simulink library "LeafEcoTronDBWLib"  (R2018a)
settings: Solver=VariableStepAuto  StartTime=0.0  StopTime=10.0  RelTol=1e-3
libraries: Simulink x17, CoderSF_BSW_Libs x3
(part 1 of 2)
settings Model: Creator=TianhuaZhang  LastModifiedBy=TianhuaZhang

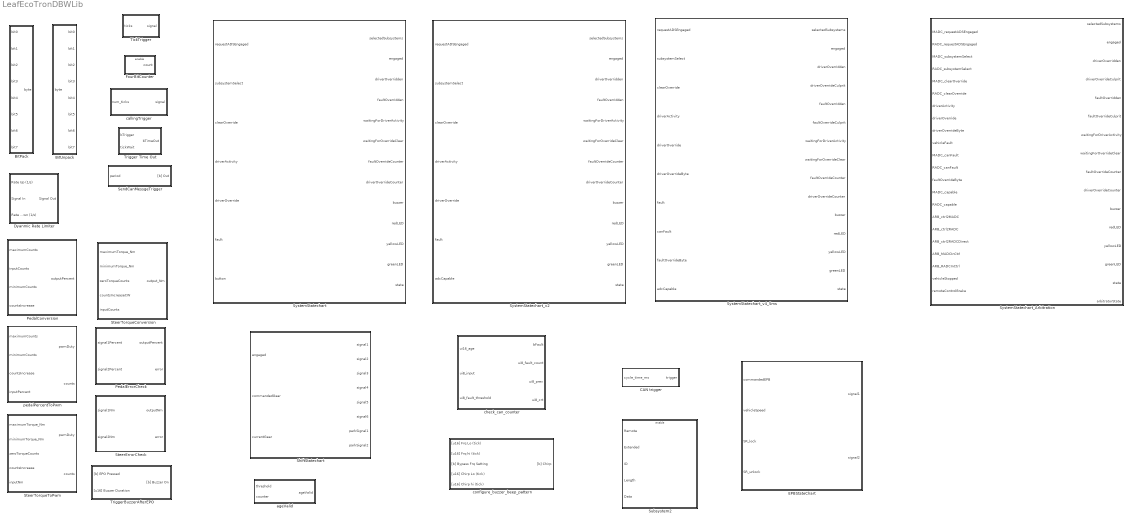
== system LeafEcoTronDBWLib ==
  BitPack : Subsystem
  BitUnpack : Subsystem
  CAN trigger : Subsystem
  Dyanmic Rate Limiter : Subsystem
  EPBStateChart : Stateflow chart  TreatAsAtomicUnit=on
  FourBitCounter : Subsystem
  PedalConversion : Subsystem
  PedalErrorCheck : Subsystem
  SendCanMessgeTrigger : Subsystem
  ShiftStatechart : Stateflow chart  TreatAsAtomicUnit=on
  SteerErrorCheck : Subsystem
  SteerTorqueConversion : Subsystem
  SteerTorqueToPwm : Subsystem
  Subsystem2 : Subsystem
  SystemStatechart : Stateflow chart  TreatAsAtomicUnit=on
  SystemStatechart_Arbitration : Stateflow chart  TreatAsAtomicUnit=on
  SystemStatechart_v2 : Stateflow chart  TreatAsAtomicUnit=on
  SystemStatechart_v4_5ms : Stateflow chart  TreatAsAtomicUnit=on
  TickTrigger : Subsystem
  Trigger Time Out : Subsystem
  TriggerBuzzerAfterEPO : Subsystem
      settings: AttributesFormatString=%<ReferenceBlock>
  ageValid : Subsystem
  callingTrigger : MATLAB Function  TreatAsAtomicUnit=on
  check_can_counter : Stateflow chart  TreatAsAtomicUnit=on
      settings: AttributesFormatString=%<ReferenceBlock>
  configure_buzzer_beep_pattern : Subsystem
      settings: AttributesFormatString=%<ReferenceBlock>
  pedalPercentToPwm : Subsystem

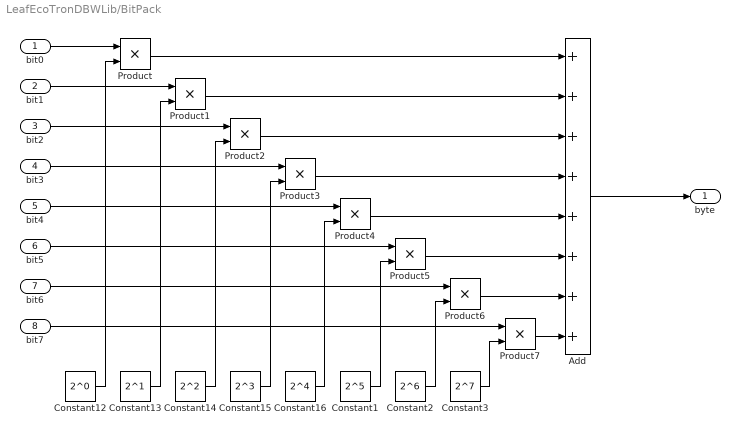
== system LeafEcoTronDBWLib/BitPack ==
  bit0 : Inport
  bit1 : Inport  Port=2
  bit2 : Inport  Port=3
  bit3 : Inport  Port=4
  bit4 : Inport  Port=5
  bit5 : Inport  Port=6
  bit6 : Inport  Port=7
  bit7 : Inport  Port=8
  Add : Sum  Inputs=++++++++  AccumDataTypeStr=uint8  OutDataTypeStr=uint8
  Constant1 : Constant  Value=2^5  OutDataTypeStr=uint8
  Constant12 : Constant  Value=2^0  OutDataTypeStr=uint8
  Constant13 : Constant  Value=2^1  OutDataTypeStr=uint8
  Constant14 : Constant  Value=2^2  OutDataTypeStr=uint8
  Constant15 : Constant  Value=2^3  OutDataTypeStr=uint8
  Constant16 : Constant  Value=2^4  OutDataTypeStr=uint8
  Constant2 : Constant  Value=2^6  OutDataTypeStr=uint8
  Constant3 : Constant  Value=2^7  OutDataTypeStr=uint8
  Product : Product  OutDataTypeStr=int16
  Product{1..7} (7 alike) : Product  OutDataTypeStr=uint8
  byte : Outport
  wires:
  Constant3/1 -> Product7/2
  Constant2/1 -> Product6/2
  Constant1/1 -> Product5/2
  Product6/1 -> Add/7
  Product5/1 -> Add/6
  bit5/1 -> Product5/1
  bit6/1 -> Product6/1
  bit7/1 -> Product7/1
  Product7/1 -> Add/8
  Product1/1 -> Add/2
  Product/1 -> Add/1
  Product4/1 -> Add/5
  Add/1 -> byte/1
  Constant16/1 -> Product4/2
  Product3/1 -> Add/4
  bit0/1 -> Product/1
  bit1/1 -> Product1/1
  bit3/1 -> Product3/1
  Constant13/1 -> Product1/2
  bit4/1 -> Product4/1
  Constant14/1 -> Product2/2
  bit2/1 -> Product2/1
  Constant15/1 -> Product3/2
  Constant12/1 -> Product/2
  Product2/1 -> Add/3

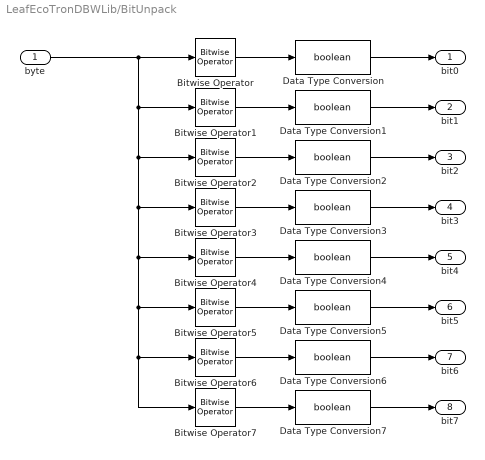
== system LeafEcoTronDBWLib/BitUnpack ==
  byte : Inport
  Bitwise Operator : Simulink/Logic and Bit Operations/Bitwise Operator  logicop=AND  UseBitMask=on  BitMask=2^0  BitMaskRealWorld=Stored Integer
      settings: SourceProductName=Simulink  SourceProductBaseCode=SL
  Bitwise Operator1 : Simulink/Logic and Bit Operations/Bitwise Operator  logicop=AND  UseBitMask=on  BitMask=2^1  BitMaskRealWorld=Stored Integer
      settings: SourceProductName=Simulink  SourceProductBaseCode=SL
  Bitwise Operator2 : Simulink/Logic and Bit Operations/Bitwise Operator  logicop=AND  UseBitMask=on  BitMask=2^2  BitMaskRealWorld=Stored Integer
      settings: SourceProductName=Simulink  SourceProductBaseCode=SL
  Bitwise Operator3 : Simulink/Logic and Bit Operations/Bitwise Operator  logicop=AND  UseBitMask=on  BitMask=2^3  BitMaskRealWorld=Stored Integer
      settings: SourceProductName=Simulink  SourceProductBaseCode=SL
  Bitwise Operator4 : Simulink/Logic and Bit Operations/Bitwise Operator  logicop=AND  UseBitMask=on  BitMask=2^4  BitMaskRealWorld=Stored Integer
      settings: SourceProductName=Simulink  SourceProductBaseCode=SL
  Bitwise Operator5 : Simulink/Logic and Bit Operations/Bitwise Operator  logicop=AND  UseBitMask=on  BitMask=2^5  BitMaskRealWorld=Stored Integer
      settings: SourceProductName=Simulink  SourceProductBaseCode=SL
  Bitwise Operator6 : Simulink/Logic and Bit Operations/Bitwise Operator  logicop=AND  UseBitMask=on  BitMask=2^6  BitMaskRealWorld=Stored Integer
      settings: SourceProductName=Simulink  SourceProductBaseCode=SL
  Bitwise Operator7 : Simulink/Logic and Bit Operations/Bitwise Operator  logicop=AND  UseBitMask=on  BitMask=2^7  BitMaskRealWorld=Stored Integer
      settings: SourceProductName=Simulink  SourceProductBaseCode=SL
  Data Type Conversion{,1..7} (8 alike) : DataTypeConversion  OutDataTypeStr=boolean
  bit0 : Outport
  bit1 : Outport  Port=2
  bit2 : Outport  Port=3
  bit3 : Outport  Port=4
  bit4 : Outport  Port=5
  bit5 : Outport  Port=6
  bit6 : Outport  Port=7
  bit7 : Outport  Port=8
  wires:
  Data Type Conversion7/1 -> bit7/1
  Data Type Conversion6/1 -> bit6/1
  Data Type Conversion5/1 -> bit5/1
  Data Type Conversion4/1 -> bit4/1
  Data Type Conversion3/1 -> bit3/1
  Data Type Conversion2/1 -> bit2/1
  Data Type Conversion1/1 -> bit1/1
  Data Type Conversion/1 -> bit0/1
  Bitwise Operator7/1 -> Data Type Conversion7/1
  Bitwise Operator6/1 -> Data Type Conversion6/1
  Bitwise Operator5/1 -> Data Type Conversion5/1
  Bitwise Operator4/1 -> Data Type Conversion4/1
  Bitwise Operator3/1 -> Data Type Conversion3/1
  Bitwise Operator2/1 -> Data Type Conversion2/1
  Bitwise Operator1/1 -> Data Type Conversion1/1
  byte/1 -> Bitwise Operator/1, Bitwise Operator7/1, Bitwise Operator6/1, Bitwise Operator5/1, Bitwise Operator4/1, Bitwise Operator3/1, Bitwise Operator2/1, Bitwise Operator1/1
  Bitwise Operator/1 -> Data Type Conversion/1

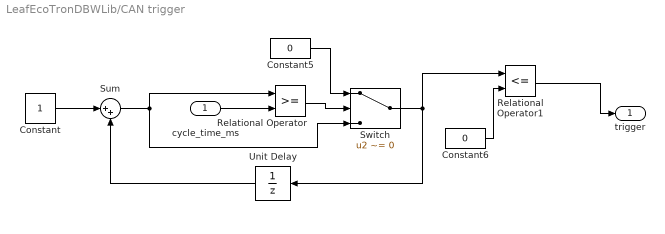
== system LeafEcoTronDBWLib/CAN trigger ==
  cycle_time_ms : Inport
  Constant : Constant  OutDataTypeStr=Inherit: Inherit via back propagation
  Constant5 : Constant  Value=0  OutDataTypeStr=Inherit: Inherit via back propagation  SampleTime=-1
  Constant6 : Constant  Value=0  OutDataTypeStr=Inherit: Inherit via back propagation  SampleTime=-1
  Relational Operator : RelationalOperator  OutDataTypeStr=boolean  RndMeth=Nearest
  Relational Operator1 : RelationalOperator  Operator=<=  OutDataTypeStr=boolean  RndMeth=Nearest
  Sum : Sum  Inputs=|++
  Switch : Switch  Criteria=u2 ~= 0
  Unit Delay : UnitDelay  SampleTime=-1
  trigger : Outport
  wires:
  cycle_time_ms/1 -> Relational Operator/2
  Relational Operator1/1 -> trigger/1
  Unit Delay/1 -> Sum/2
  Constant/1 -> Sum/1
  Relational Operator/1 -> Switch/2
  Constant5/1 -> Switch/1
  Switch/1 -> Relational Operator1/1, Unit Delay/1
  Sum/1 -> Switch/3, Relational Operator/1
  Constant6/1 -> Relational Operator1/2

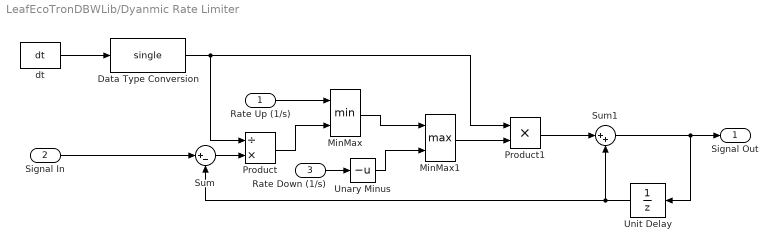
== system LeafEcoTronDBWLib/Dyanmic Rate Limiter ==
  Rate Up (1/s) : Inport
  Signal In : Inport  Port=2
  Rate Down (1/s) : Inport  Port=3
  Data Type Conversion : DataTypeConversion  OutDataTypeStr=single
  MinMax : MinMax  Inputs=2
  MinMax1 : MinMax  Function=max  Inputs=2
  Product : Product  Inputs=/*  RndMeth=Zero
  Product1 : Product  RndMeth=Zero
  Sum : Sum  Inputs=|+-
  Sum1 : Sum  Inputs=|++
  Unary Minus : UnaryMinus
  Unit Delay : UnitDelay  SampleTime=-1
  dt : CoderSF_BSW_Libs/Application Base Blocks/dt
      settings: SourceProductName=EcoCoder Blocks
  Signal Out : Outport  OutDataTypeStr=single
  wires:
  dt/1 -> Data Type Conversion/1
  Rate Up (1/s)/1 -> MinMax/1
  MinMax/1 -> MinMax1/1
  Rate Down (1/s)/1 -> Unary Minus/1
  Product/1 -> MinMax/2
  Data Type Conversion/1 -> Product/1, Product1/1
  Sum/1 -> Product/2
  MinMax1/1 -> Product1/2
  Product1/1 -> Sum1/1
  Unit Delay/1 -> Sum1/2, Sum/2
  Sum1/1 -> Unit Delay/1, Signal Out/1
  Signal In/1 -> Sum/1
  Unary Minus/1 -> MinMax1/2

== system LeafEcoTronDBWLib/FourBitCounter ==
  Enable : EnablePort
  Counter Limited : Simulink/Sources/Counter Limited  uplimit=15  tsamp=-1
      settings: SourceProductName=Simulink  SourceProductBaseCode=SL
  count : Outport
  wires:
  Counter Limited/1 -> count/1

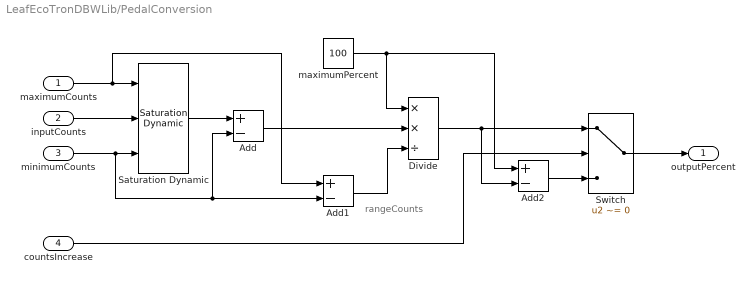
== system LeafEcoTronDBWLib/PedalConversion ==
  note: rangeCounts
  maximumCounts : Inport  OutDataTypeStr=uint16
  inputCounts : Inport  Port=2  OutDataTypeStr=uint16
  minimumCounts : Inport  Port=3  OutDataTypeStr=uint16
  countsIncrease : Inport  Port=4  OutDataTypeStr=boolean
  Add : Sum  Inputs=+-  OutDataTypeStr=single
  Add1 : Sum  Inputs=+-  OutDataTypeStr=single
  Add2 : Sum  Inputs=+-  OutDataTypeStr=single
  Divide : Product  Inputs=**/  OutDataTypeStr=single
  Saturation Dynamic : Simulink/Discontinuities/Saturation Dynamic  OutMin=[]  OutMax=[]  OutDataTypeStr=Inherit: Same as second input  OutDataType=fixdt(1, 16)  OutScaling=2^-10  DoSatur=off
      settings: SourceProductName=Simulink  SourceProductBaseCode=SL
  Switch : Switch  Criteria=u2 ~= 0
  maximumPercent : Constant  Value=100  OutDataTypeStr=single
  outputPercent : Outport
  wires:
  inputCounts/1 -> Saturation Dynamic/2
  Add1/1 -> Divide/3
  maximumPercent/1 -> Add2/1, Divide/1
  Add/1 -> Divide/2
  minimumCounts/1 -> Add/2, Add1/2, Saturation Dynamic/3
  maximumCounts/1 -> Add1/1, Saturation Dynamic/1
  Saturation Dynamic/1 -> Add/1
  Switch/1 -> outputPercent/1
  Divide/1 -> Add2/2, Switch/1
  countsIncrease/1 -> Switch/2
  Add2/1 -> Switch/3

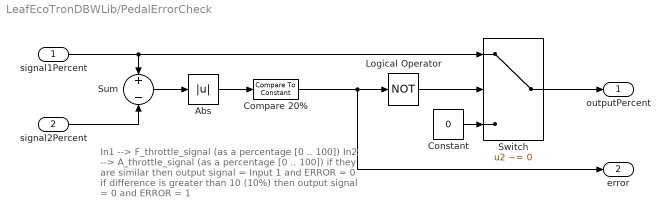
== system LeafEcoTronDBWLib/PedalErrorCheck ==
  note: In1 --> F_throttle_signal (as a percentage [0 .. 100])
      | In2 --> A_throttle_signal (as a percentage [0 .. 100])
      |
      | if they are similar then
      |     output signal = Input 1
      |     and ERROR = 0
      | if difference is greater than 10 (10%) then
      |     output signal =  0
      |     and ERROR = 1
  signal1Percent : Inport  OutDataTypeStr=single
  signal2Percent : Inport  Port=2  OutDataTypeStr=single
  Abs : Abs
  Compare 20% : Simulink/Logic and Bit Operations/Compare To Constant  relop=>=  const=20  OutDataTypeStr=boolean
      settings: SourceProductName=Simulink  SourceProductBaseCode=SL
  Constant : Constant  Value=0  OutDataTypeStr=single
  Logical Operator : Logic  Operator=NOT  AllPortsSameDT=off  OutDataTypeStr=boolean
  Sum : Sum  Inputs=+|-
  Switch : Switch  Criteria=u2 ~= 0  Threshold=0.5  OutMin=[0]  OutMax=[100]  OutDataTypeStr=single
  outputPercent : Outport  OutDataTypeStr=single
  error : Outport  Port=2  OutDataTypeStr=boolean
  wires:
  Logical Operator/1 -> Switch/2
  Constant/1 -> Switch/3
  Abs/1 -> Compare 20%/1
  Compare 20%/1 -> Logical Operator/1, error/1
  signal1Percent/1 -> Sum/1, Switch/1
  Sum/1 -> Abs/1
  signal2Percent/1 -> Sum/2
  Switch/1 -> outputPercent/1

== system LeafEcoTronDBWLib/SendCanMessgeTrigger ==
  period : Inport
  Data Type Conversion : DataTypeConversion  OutDataTypeStr=boolean
  Saturation : Saturate  UpperLimit=1000  LowerLimit=1
      settings: AttributesFormatString=[%<LowerLimit>,%<UpperLimit>]
  Terminator : Terminator
  trigger : Stateflow chart  TreatAsAtomicUnit=on
  "[b] Out" : Outport
  wires:
  trigger/2(counter) -> Terminator/1
  period/1 -> Saturation/1
  trigger/1(out) -> Data Type Conversion/1
  Data Type Conversion/1 -> "[b] Out"/1
  Saturation/1 -> trigger/1(period)

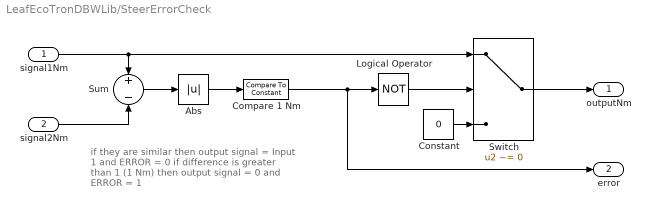
== system LeafEcoTronDBWLib/SteerErrorCheck ==
  note: if they are similar then
      |     output signal = Input 1
      |     and ERROR = 0
      | if difference is greater than 1 (1 Nm) then
      |     output signal =  0
      |     and ERROR = 1
  signal1Nm : Inport  OutDataTypeStr=single
  signal2Nm : Inport  Port=2  OutDataTypeStr=single
  Abs : Abs
  Compare 1 Nm : Simulink/Logic and Bit Operations/Compare To Constant  relop=>=  const=1  OutDataTypeStr=boolean
      settings: SourceProductName=Simulink  SourceProductBaseCode=SL
  Constant : Constant  Value=0  OutDataTypeStr=single
  Logical Operator : Logic  Operator=NOT  AllPortsSameDT=off  OutDataTypeStr=boolean
  Sum : Sum  Inputs=+|-
  Switch : Switch  Criteria=u2 ~= 0  Threshold=0.5  OutMin=[0]  OutMax=[100]  OutDataTypeStr=single
  outputNm : Outport  OutDataTypeStr=single
  error : Outport  Port=2  OutDataTypeStr=boolean
  wires:
  Logical Operator/1 -> Switch/2
  Constant/1 -> Switch/3
  Abs/1 -> Compare 1 Nm/1
  Compare 1 Nm/1 -> Logical Operator/1, error/1
  signal1Nm/1 -> Sum/1, Switch/1
  Sum/1 -> Abs/1
  signal2Nm/1 -> Sum/2
  Switch/1 -> outputNm/1

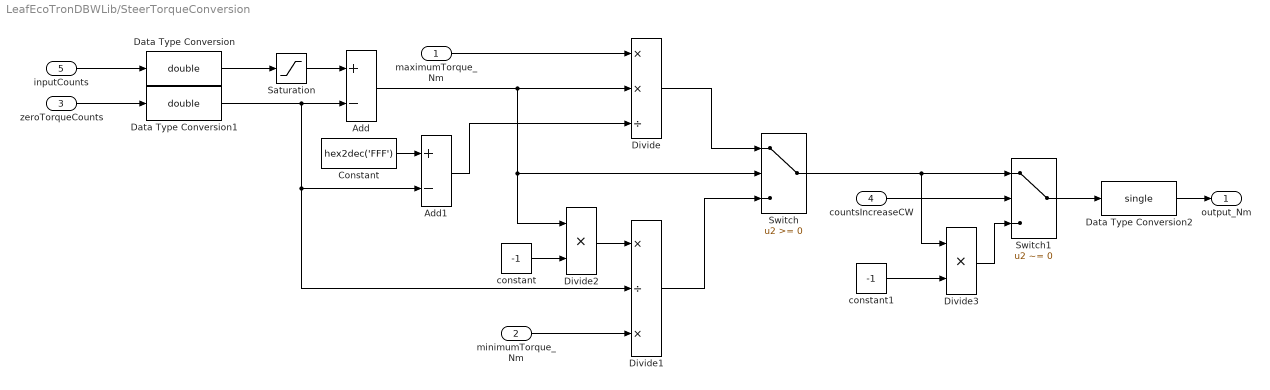
== system LeafEcoTronDBWLib/SteerTorqueConversion ==
  maximumTorque_Nm : Inport
  minimumTorque_Nm : Inport  Port=2
  zeroTorqueCounts : Inport  Port=3
  countsIncreaseCW : Inport  Port=4
  inputCounts : Inport  Port=5
  Add : Sum  Inputs=+-  OutDataTypeStr=double
  Add1 : Sum  Inputs=+-  OutDataTypeStr=double
  Constant : Constant  Value=hex2dec('FFF')  OutDataTypeStr=uint16
  Data Type Conversion : DataTypeConversion  OutDataTypeStr=double
  Data Type Conversion1 : DataTypeConversion  OutDataTypeStr=double
  Data Type Conversion2 : DataTypeConversion  OutDataTypeStr=single  LockScale=on
  Divide : Product  Inputs=**/  OutDataTypeStr=double  SaturateOnIntegerOverflow=on  RndMeth=Zero
  Divide1 : Product  Inputs=*/*  OutDataTypeStr=single  SaturateOnIntegerOverflow=on  RndMeth=Zero
  Divide2 : Product  Inputs=**  OutDataTypeStr=single  SaturateOnIntegerOverflow=on  RndMeth=Zero
  Divide3 : Product  Inputs=**  OutDataTypeStr=double  SaturateOnIntegerOverflow=on  RndMeth=Zero
  Saturation : Saturate  UpperLimit=4095  LowerLimit=0
  Switch : Switch  OutDataTypeStr=double
  Switch1 : Switch  Criteria=u2 ~= 0
  constant : Constant  Value=-1  OutDataTypeStr=single
  constant1 : Constant  Value=-1  OutDataTypeStr=single
  output_Nm : Outport
  wires:
  Data Type Conversion2/1 -> output_Nm/1
  Data Type Conversion1/1 -> Add/2, Divide1/2, Add1/2
  Data Type Conversion/1 -> Saturation/1
  Saturation/1 -> Add/1
  constant1/1 -> Divide3/2
  Divide3/1 -> Switch1/3
  countsIncreaseCW/1 -> Switch1/2
  Switch1/1 -> Data Type Conversion2/1
  Switch/1 -> Switch1/1, Divide3/1
  constant/1 -> Divide2/2
  Divide2/1 -> Divide1/1
  Divide1/1 -> Switch/3
  minimumTorque_Nm/1 -> Divide1/3
  Add1/1 -> Divide/3
  Divide/1 -> Switch/1
  maximumTorque_Nm/1 -> Divide/1
  Add/1 -> Switch/2, Divide2/1, Divide/2
  Constant/1 -> Add1/1
  zeroTorqueCounts/1 -> Data Type Conversion1/1
  inputCounts/1 -> Data Type Conversion/1

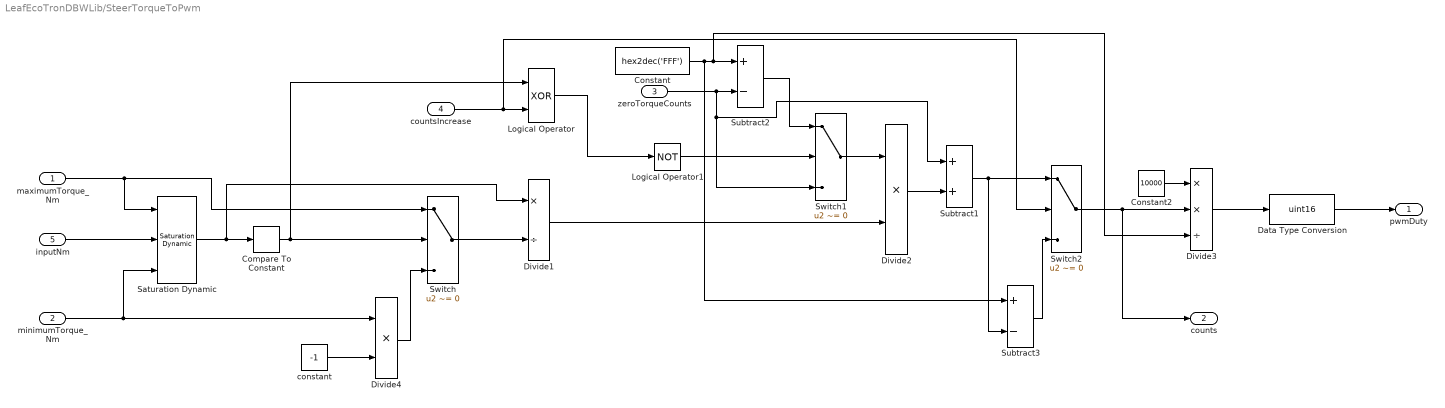
== system LeafEcoTronDBWLib/SteerTorqueToPwm ==
  maximumTorque_Nm : Inport
  minimumTorque_Nm : Inport  Port=2
  zeroTorqueCounts : Inport  Port=3
  countsIncrease : Inport  Port=4
  inputNm : Inport  Port=5
  Compare To Constant : Simulink/Logic and Bit Operations/Compare To Constant  relop=>=  const=0  OutDataTypeStr=boolean
      settings: SourceProductName=Simulink  SourceProductBaseCode=SL
  Constant : Constant  Value=hex2dec('FFF')  OutDataTypeStr=double
  Constant2 : Constant  Value=10000  OutDataTypeStr=double
  Data Type Conversion : DataTypeConversion  OutDataTypeStr=uint16
  Divide1 : Product  Inputs=*/  OutDataTypeStr=double
  Divide2 : Product  Inputs=**  OutDataTypeStr=double
  Divide3 : Product  Inputs=**/  OutDataTypeStr=double
  Divide4 : Product  Inputs=**
  Logical Operator : Logic  Operator=XOR  AllPortsSameDT=off  OutDataTypeStr=boolean
  Logical Operator1 : Logic  Operator=NOT  AllPortsSameDT=off  OutDataTypeStr=boolean
  Saturation Dynamic : Simulink/Discontinuities/Saturation Dynamic  OutMin=[]  OutMax=[]  OutDataTypeStr=Inherit: Same as second input  OutDataType=fixdt(1, 16)  OutScaling=2^-10  DoSatur=off
      settings: SourceProductName=Simulink  SourceProductBaseCode=SL
  Subtract1 : Sum  AccumDataTypeStr=double
  Subtract2 : Sum  Inputs=+-
  Subtract3 : Sum  Inputs=+-
  Switch : Switch  Criteria=u2 ~= 0  OutDataTypeStr=double
  Switch1 : Switch  Criteria=u2 ~= 0
  Switch2 : Switch  Criteria=u2 ~= 0
  constant : Constant  Value=-1  OutDataTypeStr=double
  pwmDuty : Outport
  counts : Outport  Port=2
  wires:
  Subtract3/1 -> Switch2/3
  Subtract1/1 -> Switch2/1, Subtract3/2
  Switch2/1 -> Divide3/2, counts/1
  Saturation Dynamic/1 -> Compare To Constant/1, Divide1/1
  inputNm/1 -> Saturation Dynamic/2
  Data Type Conversion/1 -> pwmDuty/1
  constant/1 -> Divide4/2
  Divide4/1 -> Switch/3
  minimumTorque_Nm/1 -> Divide4/1, Saturation Dynamic/3
  Divide2/1 -> Subtract1/2
  Logical Operator1/1 -> Switch1/2
  Logical Operator/1 -> Logical Operator1/1
  Subtract2/1 -> Switch1/1
  Compare To Constant/1 -> Logical Operator/1, Switch/2
  Divide3/1 -> Data Type Conversion/1
  Constant2/1 -> Divide3/1
  countsIncrease/1 -> Logical Operator/2, Switch2/2
  Switch1/1 -> Divide2/1
  Divide1/1 -> Divide2/2
  Switch/1 -> Divide1/2
  maximumTorque_Nm/1 -> Switch/1, Saturation Dynamic/1
  zeroTorqueCounts/1 -> Subtract2/2, Switch1/3, Subtract1/1
  Constant/1 -> Subtract2/1, Divide3/3, Subtract3/1

== system LeafEcoTronDBWLib/Subsystem2 ==
  Remote : Inport
  Extended : Inport  Port=2
  ID : Inport  Port=3
  Length : Inport  Port=4
  Data : Inport  Port=5
  Enable : EnablePort
  Transmit CAN Message : CoderSF_BSW_Libs/CAN/Transmit CAN Message  channel=CAN_B  tasktimeIndex=Task_Inherit
      settings: SourceProductName=EcoCoder Blocks
  Transmit CAN Message1 : CoderSF_BSW_Libs/CAN/Transmit CAN Message  channel=CAN_C  tasktimeIndex=Task_Inherit
      settings: SourceProductName=EcoCoder Blocks
  wires:
  Extended/1 -> Transmit CAN Message1/2, Transmit CAN Message/2
  Remote/1 -> Transmit CAN Message1/1, Transmit CAN Message/1
  Length/1 -> Transmit CAN Message1/4, Transmit CAN Message/4
  Data/1 -> Transmit CAN Message1/5, Transmit CAN Message/5
  ID/1 -> Transmit CAN Message1/3, Transmit CAN Message/3

== system LeafEcoTronDBWLib/TickTrigger ==
  ticks : Inport
  Add : Sum  OutDataTypeStr=uint8
  Compare To Zero : Simulink/Logic and Bit Operations/Compare To Zero  relop===  OutDataTypeStr=boolean
      settings: SourceProductName=Simulink  SourceProductBaseCode=SL
  Constant2 : Constant
  Memory : Memory  InheritSampleTime=on
  Mod : Math  Operator=mod  SaturateOnIntegerOverflow=on
  signal : Outport  OutDataTypeStr=boolean
  wires:
  Compare To Zero/1 -> signal/1
  Add/1 -> Mod/1
  Memory/1 -> Add/1
  Constant2/1 -> Add/2
  ticks/1 -> Mod/2
  Mod/1 -> Memory/1, Compare To Zero/1

== system LeafEcoTronDBWLib/Trigger Time Out ==
  note: -Once the bTrigger signal is high, program starts counting and set bTimeOut to high when it exceeds the tickWati
      | -bTimeOut resets as soon as bTrigger resets
  bTrigger : Inport
  tickWait : Inport  Port=2
  Constant : Constant  Value=0  OutDataTypeStr=single
      settings: AttributesFormatString=%<OutDataTypeStr>
  IC1 : InitialCondition
  Increment Real World1 : Simulink/Additional Math & Discrete/Additional Math: Increment - Decrement/Increment Real World
      settings: SourceProductName=Simulink  SourceProductBaseCode=SL
  Memory1 : Memory  InheritSampleTime=on
  Relational Operator1 : RelationalOperator  Operator=>  OutDataTypeStr=boolean  RndMeth=Nearest
  Switch1 : Switch  Criteria=u2 > Threshold
  bTimeOut : Outport
  wires:
  Relational Operator1/1 -> bTimeOut/1
  tickWait/1 -> Relational Operator1/2
  Memory1/1 -> IC1/1, Relational Operator1/1
  Switch1/1 -> Memory1/1
  Increment Real World1/1 -> Switch1/1
  IC1/1 -> Increment Real World1/1
  bTrigger/1 -> Switch1/2
  Constant/1 -> Switch1/3

== system LeafEcoTronDBWLib/TriggerBuzzerAfterEPO ==
  "[b] EPO Pressed" : Inport
  "[u16] Buzzer Duration" : Inport  Port=2
  Detect Increase : Simulink/Logic and Bit Operations/Detect Increase  vinit=0.0  OutDataTypeStr=boolean
      settings: SourceProductName=Simulink  SourceProductBaseCode=SL
  trigger_buzzer_after_epo : Stateflow chart  TreatAsAtomicUnit=on
  "[b] Buzzer On" : Outport
  wires:
  Detect Increase/1 -> trigger_buzzer_after_epo/1(bEPO_rise)
  "[b] EPO Pressed"/1 -> Detect Increase/1
  "[u16] Buzzer Duration"/1 -> trigger_buzzer_after_epo/2(tick_duration)
  trigger_buzzer_after_epo/1(bBuzzer) -> "[b] Buzzer On"/1

== system LeafEcoTronDBWLib/ageValid ==
  threshold : Inport
  counter : Inport  Port=2
  Data Type Conversion : DataTypeConversion  OutDataTypeStr=uint16
  Data Type Conversion2 : DataTypeConversion  OutDataTypeStr=boolean
  Delay : Delay  DelayLength=1
  Relational Operator : RelationalOperator  Operator=~=  OutDataTypeStr=boolean  RndMeth=Nearest
  trigger : Stateflow chart  AncestorBlock=LeafDbWLibrary/SendCanMessgeTrigger/trigger  TreatAsAtomicUnit=on
  ageValid : Outport  OutDataTypeStr=boolean
  wires:
  Delay/1 -> Relational Operator/1
  Relational Operator/1 -> trigger/2(update)
  threshold/1 -> Data Type Conversion/1
  trigger/1(ageValid) -> Data Type Conversion2/1
  Data Type Conversion/1 -> trigger/1(threshold)
  counter/1 -> Delay/1, Relational Operator/2
  Data Type Conversion2/1 -> ageValid/1

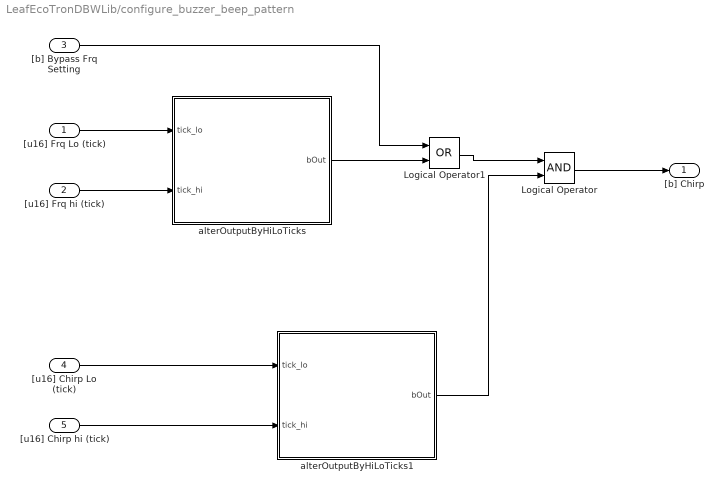
== system LeafEcoTronDBWLib/configure_buzzer_beep_pattern ==
  "[u16] Frq Lo (tick)" : Inport
  "[u16] Frq hi (tick)" : Inport  Port=2
  "[b] Bypass Frq Setting" : Inport  Port=3
  "[u16] Chirp Lo (tick)" : Inport  Port=4
  "[u16] Chirp hi (tick)" : Inport  Port=5
  Logical Operator : Logic  AllPortsSameDT=off  OutDataTypeStr=boolean
  Logical Operator1 : Logic  Operator=OR  AllPortsSameDT=off  OutDataTypeStr=boolean
  alterOutputByHiLoTicks : Stateflow chart  TreatAsAtomicUnit=on
  alterOutputByHiLoTicks1 : Stateflow chart  TreatAsAtomicUnit=on
  "[b] Chirp" : Outport
  wires:
  "[u16] Frq hi (tick)"/1 -> alterOutputByHiLoTicks/2(tick_hi)
  "[u16] Frq Lo (tick)"/1 -> alterOutputByHiLoTicks/1(tick_lo)
  "[u16] Chirp hi (tick)"/1 -> alterOutputByHiLoTicks1/2(tick_hi)
  "[u16] Chirp Lo (tick)"/1 -> alterOutputByHiLoTicks1/1(tick_lo)
  Logical Operator1/1 -> Logical Operator/1
  alterOutputByHiLoTicks1/1(bOut) -> Logical Operator/2
  Logical Operator/1 -> "[b] Chirp"/1
  alterOutputByHiLoTicks/1(bOut) -> Logical Operator1/2
  "[b] Bypass Frq Setting"/1 -> Logical Operator1/1

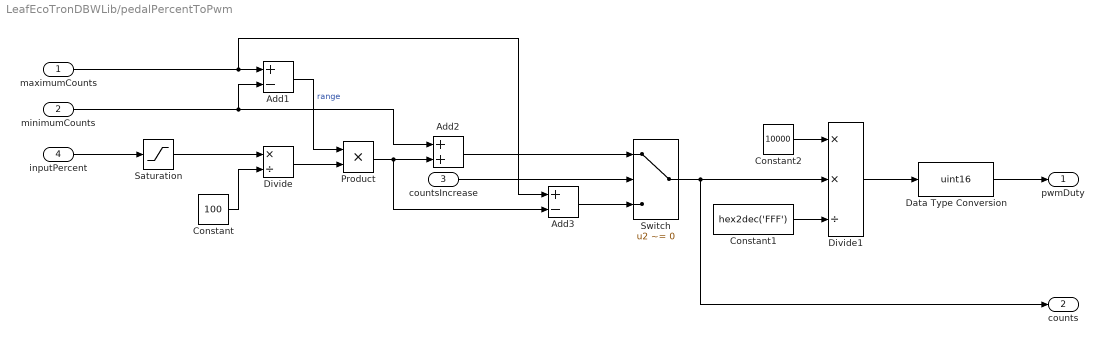
== system LeafEcoTronDBWLib/pedalPercentToPwm ==
  maximumCounts : Inport
  minimumCounts : Inport  Port=2
  countsIncrease : Inport  Port=3
  inputPercent : Inport  Port=4
  Add1 : Sum  Inputs=+-  OutDataTypeStr=single
  Add2 : Sum  OutDataTypeStr=single
  Add3 : Sum  Inputs=+-  OutDataTypeStr=single
  Constant : Constant  Value=100  OutDataTypeStr=single
  Constant1 : Constant  Value=hex2dec('FFF')  OutDataTypeStr=single
  Constant2 : Constant  Value=10000  OutDataTypeStr=single
  Data Type Conversion : DataTypeConversion  OutDataTypeStr=uint16
  Divide : Product  Inputs=*/
  Divide1 : Product  Inputs=**/  OutDataTypeStr=single
  Product : Product
  Saturation : Saturate  UpperLimit=100.0  LowerLimit=0.0
  Switch : Switch  Criteria=u2 ~= 0
  pwmDuty : Outport
  counts : Outport  Port=2
  wires:
  Divide/1 -> Product/2
  Saturation/1 -> Divide/1
  Add2/1 -> Switch/1
  Add3/1 -> Switch/3
  countsIncrease/1 -> Switch/2
  Constant/1 -> Divide/2
  Divide1/1 -> Data Type Conversion/1
  maximumCounts/1 -> Add1/1, Add3/1
  minimumCounts/1 -> Add2/1, Add1/2
  inputPercent/1 -> Saturation/1
  Add1/1 -> Product/1  "range"
  Product/1 -> Add2/2, Add3/2
  Switch/1 -> counts/1, Divide1/2
  Constant2/1 -> Divide1/1
  Constant1/1 -> Divide1/3
  Data Type Conversion/1 -> pwmDuty/1

== stateflow chart LeafEcoTronDBWLib/SystemStatechart_v2 ==
  state Initializing
    entry:
    state = SystemState.INITIALIZING;
    engaged = false;
    selectedSubsystems = subsystemSelect;
    driverOverridden = false;
    faultOverridden = false;
    faultOverrideCounter = uint8(0);
    driverOverrideCounter = uint8(0);
    waitingForDriverActivity = false;
    waitingForOverrideClear = false;
    buzzer = false;
    state LedsOff
      entry:
      redLED = LEDState.LED_OFF;
      yellowLED = LEDState.LED_OFF;
      greenLED = LEDState.LED_OFF;
    state RedLedOn
      entry:
      redLED = LEDState.LED_ON;
      yellowLED = LEDState.LED_OFF;
      greenLED = LEDState.LED_OFF;
    state YellowLedOn
      entry:
      redLED = LEDState.LED_OFF;
      yellowLED = LEDState.LED_ON;
      greenLED = LEDState.LED_OFF;
    state GreenLedOn
      entry:
      redLED = LEDState.LED_OFF;
      yellowLED = LEDState.LED_OFF;
      greenLED = LEDState.LED_ON;
    state AllLedsOn
      entry:
      redLED = LEDState.LED_ON;
      yellowLED = LEDState.LED_ON;
      greenLED = LEDState.LED_ON;
    (default) -> LedsOff
    LedsOff -> RedLedOn : after(1000, tick)
    RedLedOn -> YellowLedOn : after(1000, tick)
    YellowLedOn -> GreenLedOn : after(1000, tick)
    GreenLedOn -> AllLedsOn : after(1000, tick)
  state ADSDisengaged
    state PreOperational
      during: selectedSubsystems = subsystemSelect;
      state LLC [parallel]
        settings: executionOrder=1
        state LLCNotReady
          entry:
          state = SystemState.NOT_READY;
          redLED = LEDState.LED_ON;
          yellowLED = LEDState.LED_OFF;
        state LLCReady
          entry:
          state = SystemState.READY;
          redLED = LEDState.LED_OFF;
          yellowLED = LEDState.LED_ON;
        (default) -> LLCNotReady
        LLCReady -> LLCNotReady : [fault]
        LLCNotReady -> LLCReady : [~fault]
      state ADC [parallel]
        settings: executionOrder=2
        state ADCNotReady
          entry:
          greenLED = LEDState.LED_OFF;
        state ADCReady
          entry:
          greenLED = LEDState.LED_SLOW_PULSE;
        (default) -> ADCNotReady
        ADCReady -> ADCNotReady : [~adcCapable]
        ADCNotReady -> ADCReady : [adcCapable]
    state FaultOverridden
      entry:
      state = SystemState.FAULT_OVERRIDDEN;
      engaged = false;
      faultOverridden = true;
      exit:
      faultOverridden = false;
      state WaitingForADC
        entry:
        waitingForOverrideClear = true;
        redLED = LEDState.LED_ON;
        yellowLED = LEDState.LED_OFF;
        greenLED = LEDState.LED_OFF;
        exit:
        waitingForOverrideClear = false;
      state AlertingDriver
        entry:
        buzzer = true;
        redLED = LEDState.LED_FAST_PULSE;
        yellowLED = LEDState.LED_FAST_PULSE;
        greenLED = LEDState.LED_FAST_PULSE;
      state WaitingForDriverActivity
        entry:
        waitingForDriverActivity = true;
        exit:
        buzzer = false;
        waitingForDriverActivity = false;
      ADSDisengaged.FaultOverridden.WaitingForDriverActivity -> ADSDisengaged.FaultOverridden.WaitingForADC : [driverActivity || selectedSubsystems == 1 || selectedSubsystems == 4 || selectedSubsystems == 5]
      ADSDisengaged.FaultOverridden.AlertingDriver -> ADSDisengaged.FaultOverridden.WaitingForDriverActivity : after(500,tick)
    state WaitingForDriverActivity
      entry:
      waitingForDriverActivity = true;
      exit:
      buzzer = false;
      waitingForDriverActivity = false;
    state DriverOverridden
      entry:
      state = SystemState.DRIVER_OVERRIDDEN;
      engaged = false;
      driverOverridden = true;
      exit:
      driverOverridden = false;
      state AlertingDriver
        entry:
        buzzer = true;
        redLED = LEDState.LED_FAST_PULSE;
        yellowLED = LEDState.LED_FAST_PULSE;
        greenLED = LEDState.LED_FAST_PULSE;
        exit:
        buzzer = false;
      state WaitingForADC
        entry:
        waitingForOverrideClear = true;
        redLED = LEDState.LED_ON;
        yellowLED = LEDState.LED_OFF;
        greenLED = LEDState.LED_OFF;
        exit:
        waitingForOverrideClear = false;
      ADSDisengaged.DriverOverridden.AlertingDriver -> ADSDisengaged.DriverOverridden.WaitingForADC : after(500,tick)
    state ADSRelinquishWarning
      entry:
      state = SystemState.ADS_RELINQUISH_WARNING;
      engaged = false;
      buzzer = true;
      redLED = LEDState.LED_FAST_PULSE;
      yellowLED = LEDState.LED_FAST_PULSE;
      greenLED = LEDState.LED_FAST_PULSE;
    ADSDisengaged.DriverOverridden.WaitingForADC -> PreOperational : [clearOverride && ~requestADSEngaged]
    ADSDisengaged.FaultOverridden.WaitingForADC -> PreOperational : [clearOverride && ~requestADSEngaged]
    ADSDisengaged.WaitingForDriverActivity -> PreOperational : [driverActivity || selectedSubsystems == 1 || selectedSubsystems == 4 || selectedSubsystems == 5]
    ADSRelinquishWarning -> ADSDisengaged.WaitingForDriverActivity : after(500,tick)
  state ADSEngaged
    entry:
    state = SystemState.ADS_ENGAGED;
    engaged = true;
    selectedSubsystems = subsystemSelect;
    redLED = LEDState.LED_OFF;
    yellowLED = LEDState.LED_OFF;
    greenLED = LEDState.LED_ON;
  (default) -> Initializing
  AllLedsOn -> PreOperational : after(1000, tick)
  PreOperational -> ADSEngaged : [~fault && adcCapable && requestADSEngaged && (selectedSubsystems ~= 0)]
  ADSEngaged -> ADSDisengaged.FaultOverridden.AlertingDriver [order 1] : [fault]{faultOverrideCounter = faultOverrideCounter + 1;}
  ADSEngaged -> ADSDisengaged.DriverOverridden.AlertingDriver [order 3] : [driverOverride]{driverOverrideCounter = driverOverrideCounter + 1;}
  ADSEngaged -> ADSRelinquishWarning [order 2] : [~requestADSEngaged]
  data: selectedSubsystems output uint8; engaged output boolean; driverOverridden output boolean; faultOverridden output boolean; waitingForDriverActivity output boolean; waitingForOverrideClear output boolean; faultOverrideCounter output uint8; driverOverrideCounter output uint8; requestADSEngaged input boolean; subsystemSelect input uint8; clearOverride input boolean; buzzer output boolean; driverActivity input boolean; driverOverride input boolean; fault input boolean; adcCapable input boolean; redLED output; yellowLED output; greenLED output; state output

== stateflow chart LeafEcoTronDBWLib/ageValid/trigger ==
  state ini
    entry:
    ageValid = false;
  state wait
  state age_valid
    entry:
    ageValid = true;
  state age_invalid
    entry:
    ageValid = false;
  (default) -> ini
  ini -> age_valid : [update==true]
  age_valid -> wait : [update == false]
  wait -> age_invalid [order 2] : after(threshold, tick)
  wait -> age_valid [order 1] : [update == true]
  age_invalid -> age_valid : [update == true]
  data: ageValid output boolean; counter local uint16; threshold input uint16; update input boolean

== stateflow chart LeafEcoTronDBWLib/SystemStatechart ==
  state Initializing
    entry:
    state = SystemState.INITIALIZING;
    engaged = false;
    selectedSubsystems = subsystemSelect;
    driverOverridden = false;
    faultOverridden = false;
    faultOverrideCounter = uint8(0);
    driverOverrideCounter = uint8(0);
    waitingForDriverActivity = false;
    waitingForOverrideClear = false;
    buzzer = false;
    redLED = LEDState.LED_OFF;
    yellowLED = LEDState.LED_OFF;
    greenLED = LEDState.LED_OFF;
  state ADSDisengaged
    state NotReady
      entry:
      state = SystemState.NOT_READY;
      redLED = LEDState.LED_ON;
      yellowLED = LEDState.LED_OFF;
      greenLED = LEDState.LED_OFF;
      during:
      selectedSubsystems = subsystemSelect;
    state FaultOverridden
      entry:
      state = SystemState.FAULT_OVERRIDDEN;
      engaged = false;
      faultOverridden = true;
      exit:
      faultOverridden = false;
      state WaitingForADC
        entry:
        waitingForOverrideClear = true;
        exit:
        waitingForOverrideClear = false;
      state AlertingDriver
        entry:
        buzzer = true;
        redLED = LEDState.LED_FAST_PULSE;
        yellowLED = LEDState.LED_FAST_PULSE;
        greenLED = LEDState.LED_FAST_PULSE;
      state WaitingForDriverActivity
        entry:
        waitingForDriverActivity = true;
        exit:
        buzzer = false;
        waitingForDriverActivity = false;
      ADSDisengaged.FaultOverridden.WaitingForDriverActivity -> ADSDisengaged.FaultOverridden.WaitingForADC : [driverActivity]
      ADSDisengaged.FaultOverridden.AlertingDriver -> ADSDisengaged.FaultOverridden.WaitingForDriverActivity : after(500,tick)
    state WaitingForDriverActivity
      entry:
      waitingForDriverActivity = true;
      exit:
      buzzer = false;
      waitingForDriverActivity = false;
    state Ready
      entry:
      state = SystemState.READY;
      redLED = LEDState.LED_OFF;
      yellowLED = LEDState.LED_ON;
      greenLED = LEDState.LED_OFF;
      during:
      selectedSubsystems = subsystemSelect;
    state DriverOverridden
      entry:
      state = SystemState.DRIVER_OVERRIDDEN;
      engaged = false;
      driverOverridden = true;
      exit:
      driverOverridden = false;
      state AlertingDriver
        entry:
        buzzer = true;
        redLED = LEDState.LED_FAST_PULSE;
        yellowLED = LEDState.LED_FAST_PULSE;
        greenLED = LEDState.LED_FAST_PULSE;
        exit:
        buzzer = false;
      state WaitingForADC
        entry:
        waitingForOverrideClear = true;
        exit:
        waitingForOverrideClear = false;
      ADSDisengaged.DriverOverridden.AlertingDriver -> ADSDisengaged.DriverOverridden.WaitingForADC : after(500,tick)
    state ADSRelinquishWarning
      entry:
      state = SystemState.ADS_RELINQUISH_WARNING;
      engaged = false;
      buzzer = true;
      redLED = LEDState.LED_FAST_PULSE;
      yellowLED = LEDState.LED_FAST_PULSE;
      greenLED = LEDState.LED_FAST_PULSE;
    ADSDisengaged.FaultOverridden.WaitingForADC -> NotReady : [clearOverride && ~requestADSEngaged]
    ADSDisengaged.DriverOverridden.WaitingForADC -> NotReady : [clearOverride && ~requestADSEngaged]
    ADSDisengaged.WaitingForDriverActivity -> NotReady : [driverActivity]
    Ready -> NotReady [order 1] : [fault]
    NotReady -> Ready : [~fault]
    ADSRelinquishWarning -> ADSDisengaged.WaitingForDriverActivity : after(500,tick)
  state ADSEngaged
    entry:
    state = SystemState.ADS_ENGAGED;
    engaged = true;
    selectedSubsystems = subsystemSelect;
    redLED = LEDState.LED_OFF;
    yellowLED = LEDState.LED_OFF;
    greenLED = LEDState.LED_ON;
  (default) -> Initializing
  Initializing -> NotReady
  Ready -> ADSEngaged [order 2] : [requestADSEngaged]
  ADSEngaged -> ADSDisengaged.FaultOverridden.AlertingDriver [order 1] : [fault]{faultOverrideCounter = faultOverrideCounter + 1;}
  ADSEngaged -> ADSDisengaged.DriverOverridden.AlertingDriver [order 3] : [driverOverride]{driverOverrideCounter = driverOverrideCounter + 1;}
  ADSEngaged -> ADSRelinquishWarning [order 2] : [~requestADSEngaged]
  data: selectedSubsystems output uint8; engaged output boolean; driverOverridden output boolean; faultOverridden output boolean; waitingForDriverActivity output boolean; waitingForOverrideClear output boolean; faultOverrideCounter output uint8; driverOverrideCounter output uint8; requestADSEngaged input boolean; subsystemSelect input uint8; clearOverride input boolean; buzzer output boolean; driverActivity input boolean; driverOverride input boolean; fault input boolean; button input boolean; redLED output; yellowLED output; greenLED output; state output

== stateflow chart LeafEcoTronDBWLib/SendCanMessgeTrigger/trigger ==
  state ini
    entry:
    out = 0;
    counter = 0;
  state increase
    during:
    counter = counter + 1;
    exit:
    out = 1;
  state decrease
    during:
    counter = counter - 1;
    exit:
    out = 0;
  (default) -> ini
  ini -> increase
  decrease -> increase : [counter <= 0]
  increase -> decrease : [counter >= period - 1]
  data: period input; out output; counter output

== matlab function LeafEcoTronDBWLib/callingTrigger ==
  data: num_ticks input; signal output
function signal = callingTrigger(num_ticks)
signal = false;
signal = coder.ceval('trigger', num_ticks);

== stateflow chart LeafEcoTronDBWLib/SystemStatechart_v4_5ms ==
  state Initializing
    entry:
    state = SystemState.INITIALIZING;
    engaged = false;
    selectedSubsystems = subsystemSelect;
    driverOverridden = false;
    driverOverrideCulprit = uint8(0);
    faultOverridden = false;
    faultOverrideCulprit = uint8(0);
    faultOverrideCounter = uint8(0);
    driverOverrideCounter = uint8(0);
    waitingForDriverActivity = false;
    waitingForOverrideClear = false;
    buzzer = false;
    state LedsOff
      entry:
      redLED = LEDState.LED_OFF;
      yellowLED = LEDState.LED_OFF;
      greenLED = LEDState.LED_OFF;
    state RedLedOn
      entry:
      redLED = LEDState.LED_ON;
      yellowLED = LEDState.LED_OFF;
      greenLED = LEDState.LED_OFF;
    state YellowLedOn
      entry:
      redLED = LEDState.LED_OFF;
      yellowLED = LEDState.LED_ON;
      greenLED = LEDState.LED_OFF;
    state GreenLedOn
      entry:
      redLED = LEDState.LED_OFF;
      yellowLED = LEDState.LED_OFF;
      greenLED = LEDState.LED_ON;
    state AllLedsOn
      entry:
      redLED = LEDState.LED_ON;
      yellowLED = LEDState.LED_ON;
      greenLED = LEDState.LED_ON;
    (default) -> LedsOff
    LedsOff -> RedLedOn : after(1000/5, tick)
    RedLedOn -> YellowLedOn : after(1000/5, tick)
    YellowLedOn -> GreenLedOn : after(1000/5, tick)
    GreenLedOn -> AllLedsOn : after(1000/5, tick)
  state ADSDisengaged
    state PreOperational
      entry: driverOverrideCulprit = uint8(0); faultOverrideCulprit = uint8(0);
      during: selectedSubsystems = subsystemSelect;
      state LLC [parallel]
        settings: executionOrder=1
        state LLCNotReady
          entry:
          state = SystemState.NOT_READY;
          redLED = LEDState.LED_ON;
          yellowLED = LEDState.LED_OFF;
        state LLCReady
          entry:
          state = SystemState.READY;
          redLED = LEDState.LED_OFF;
          yellowLED = LEDState.LED_ON;
        (default) -> LLCNotReady
        LLCReady -> LLCNotReady : [fault || ~adcCapable]
        LLCNotReady -> LLCReady : [~fault && adcCapable]
      state ADC [parallel]
        settings: executionOrder=2
        state ADCNotReady
          entry:
          greenLED = LEDState.LED_OFF;
        state ADCReady
          entry:
          greenLED = LEDState.LED_SLOW_PULSE;
        (default) -> ADCNotReady
        ADCReady -> ADCNotReady : [~adcCapable]
        ADCNotReady -> ADCReady : [adcCapable]
    state FaultOverridden
      entry:
      state = SystemState.FAULT_OVERRIDDEN;
      engaged = false;
      faultOverridden = true;
      exit:
      faultOverridden = false;
      state WaitingForADC
        entry:
        waitingForOverrideClear = true;
        redLED = LEDState.LED_ON;
        yellowLED = LEDState.LED_OFF;
        greenLED = LEDState.LED_OFF;
        exit:
        waitingForOverrideClear = false;
      state AlertingDriver
        entry:
        buzzer = true;
        redLED = LEDState.LED_FAST_PULSE;
        yellowLED = LEDState.LED_FAST_PULSE;
        greenLED = LEDState.LED_FAST_PULSE;
      state WaitingForDriverActivity
        entry:
        waitingForDriverActivity = true;
        exit:
        buzzer = false;
        waitingForDriverActivity = false;
      ADSDisengaged.FaultOverridden.WaitingForDriverActivity -> ADSDisengaged.FaultOverridden.WaitingForADC : [driverActivity || selectedSubsystems == 1 || selectedSubsystems == 4 || selectedSubsystems == 5]
      ADSDisengaged.FaultOverridden.AlertingDriver -> ADSDisengaged.FaultOverridden.WaitingForDriverActivity : after(500/5,tick)
    state WaitingForDriverActivity
      entry:
      waitingForDriverActivity = true;
      exit:
      buzzer = false;
      waitingForDriverActivity = false;
    state DriverOverridden
      entry:
      state = SystemState.DRIVER_OVERRIDDEN;
      engaged = false;
      driverOverridden = true;
      exit:
      driverOverridden = false;
      state AlertingDriver
        entry:
        buzzer = true;
        redLED = LEDState.LED_FAST_PULSE;
        yellowLED = LEDState.LED_FAST_PULSE;
        greenLED = LEDState.LED_FAST_PULSE;
        exit:
        buzzer = false;
      state WaitingForADC
        entry:
        waitingForOverrideClear = true;
        redLED = LEDState.LED_ON;
        yellowLED = LEDState.LED_OFF;
        greenLED = LEDState.LED_OFF;
        exit:
        waitingForOverrideClear = false;
      ADSDisengaged.DriverOverridden.AlertingDriver -> ADSDisengaged.DriverOverridden.WaitingForADC : after(500/5,tick)
    state ADSRelinquishWarning
      entry:
      state = SystemState.ADS_RELINQUISH_WARNING;
      engaged = false;
      buzzer = true;
      redLED = LEDState.LED_FAST_PULSE;
      yellowLED = LEDState.LED_FAST_PULSE;
      greenLED = LEDState.LED_FAST_PULSE;
    ADSDisengaged.DriverOverridden.WaitingForADC -> PreOperational : [clearOverride && ~requestADSEngaged]
    ADSDisengaged.FaultOverridden.WaitingForADC -> PreOperational : [clearOverride && ~requestADSEngaged]
    ADSDisengaged.WaitingForDriverActivity -> PreOperational : [driverActivity || selectedSubsystems == 1 || selectedSubsystems == 4 || selectedSubsystems == 5]
    ADSRelinquishWarning -> ADSDisengaged.WaitingForDriverActivity : after(500/5,tick)
  state ADSEngaged
    entry:
    state = SystemState.ADS_ENGAGED;
    engaged = true;
    selectedSubsystems = subsystemSelect;
    redLED = LEDState.LED_OFF;
    yellowLED = LEDState.LED_OFF;
    greenLED = LEDState.LED_ON;
    exit:
    driverOverrideCulprit = driverOverrideByte;
    faultOverrideCulprit = faultOverrideByte;
    state RedLightOff
      entry:
      redLED = LEDState.LED_OFF;
    state RedLightOn
      entry:
      redLED = LEDState.LED_FAST_PULSE;
    (default) -> RedLightOff
    RedLightOn -> RedLightOff : [adcCapable]
    RedLightOff -> RedLightOn : [~adcCapable]
  (default) -> Initializing
  AllLedsOn -> PreOperational : after(1000/5, tick)
  PreOperational -> ADSEngaged : [~(fault || canFault) && adcCapable && requestADSEngaged && (selectedSubsystems ~= 0)]
  ADSEngaged -> ADSDisengaged.FaultOverridden.AlertingDriver [order 1] : [fault || canFault]{faultOverrideCounter = faultOverrideCounter + 1;}
  ADSEngaged -> ADSDisengaged.DriverOverridden.AlertingDriver [order 3] : [driverOverride]{driverOverrideCounter = driverOverrideCounter + 1;}
  ADSEngaged -> ADSRelinquishWarning [order 2] : [~requestADSEngaged]
  data: selectedSubsystems output uint8; engaged output boolean; driverOverridden output boolean; driverOverrideCulprit output uint8; faultOverridden output boolean; faultOverrideCulprit output uint8; waitingForDriverActivity output boolean; waitingForOverrideClear output boolean; faultOverrideCounter output uint8; driverOverrideCounter output uint8; requestADSEngaged input boolean; subsystemSelect input uint8; clearOverride input boolean; buzzer output boolean; driverActivity input boolean; driverOverride input boolean; driverOverrideByte input uint8; fault input boolean; canFault input boolean; faultOverrideByte input uint8; adcCapable input boolean; redLED output; yellowLED output; greenLED output; state output

== stateflow chart LeafEcoTronDBWLib/check_can_counter ==
  state ini
    entry:
    ui8_fault_count = uint8(0);
    ui8_prev = uint8(0);
    ui8_crt = uint8(0);
    bFault = false;
  state refresh_counter
    entry:
    ui8_prev = ui8_crt;
    ui8_crt = ui8_input;
  state counter_is_invalid
    entry:
    ui8_fault_count = ui8_fault_count + uint8(1);
    bFault = ui8_fault_count > ui8_fault_threshold;
    state done
    state wait
    (default) -> counter_is_invalid.wait
    counter_is_invalid.wait -> counter_is_invalid.done : after(1,tick)
  state counter_is_valid
    entry:
    ui8_fault_count = uint8(0);
    bFault = false;
    state done
    state wait
    (default) -> counter_is_valid.wait
    counter_is_valid.wait -> counter_is_valid.done : after(1,tick)
  (default) -> ini
  counter_is_valid -> ini : [ui8_crt == 0]
  counter_is_invalid -> ini : [ui8_crt == 0]
  ini -> refresh_counter : [ui16_age == 0]
  refresh_counter -> counter_is_invalid [order 2] : [(ui8_crt ~= 1 && ui8_crt ~= ui8_prev + 1) || ...
      | (ui8_crt == 1 && ui8_prev ~= 255)]
  counter_is_valid.done -> refresh_counter : [ui16_age == 0]
  refresh_counter -> counter_is_valid [order 1] : [(ui8_crt ~= 1 && ui8_crt == ui8_prev + 1) || ...
      | (ui8_crt == 1 && ui8_prev == 255)]
  counter_is_invalid.done -> refresh_counter : [ui16_age == 0]
  data: ui16_age input; ui8_input input; ui8_fault_threshold input; bFault output; ui8_fault_count output; ui8_prev output; ui8_crt output

== stateflow chart LeafEcoTronDBWLib/TriggerBuzzerAfterEPO/trigger_buzzer_after_epo ==
  state buzzer_off
    entry:
    bBuzzer = false;
  state buzzer_on
    entry:
    bBuzzer = true;
  (default) -> buzzer_off
  buzzer_off -> buzzer_on : [bEPO_rise == true]
  buzzer_on -> buzzer_off : after(tick_duration,tick)
  data: bEPO_rise input; tick_duration input; bBuzzer output

== stateflow chart LeafEcoTronDBWLib/configure_buzzer_beep_pattern/alterOutputByHiLoTicks ==
  state lo
    entry:
    bOut = false;
  state hi
    entry:
    bOut = true;
  (default) -> lo
  hi -> lo : after(tick_hi, tick)
  lo -> hi : after(tick_lo, tick)
  data: tick_lo input; tick_hi input; bOut output

== stateflow chart LeafEcoTronDBWLib/configure_buzzer_beep_pattern/alterOutputByHiLoTicks1 ==
  state lo
    entry:
    bOut = false;
  state hi
    entry:
    bOut = true;
  (default) -> lo
  hi -> lo : after(tick_hi, tick)
  lo -> hi : after(tick_lo, tick)
  data: tick_lo input; tick_hi input; bOut output

== stateflow chart LeafEcoTronDBWLib/ShiftStatechart ==
  state Home
    entry:
    signal1 = false;
    signal2 = false;
    signal3 = true;
    signal4 = false;
    signal5 = false;
    signal6 = true;
    parkSignal1 = false;
    parkSignal2 = true;
    state Wait
    state Ready
    (default) -> Wait
    Wait -> Ready : after(1250, tick)
  state Shifting
  (default) -> Home
  (junction 17) -> Shifting : after(1000, tick)
  (junction 15) -> (junction 17) [order 2] : [commandedGear == GearState.GEAR_NEUTRAL]
      | {signal2 = true; signal3 = true; signal4 = true; signal6 = false;}
  (junction 20) -> (junction 43) : after(300, tick)
      | {parkSignal1 = false; parkSignal2 = true;}
  (junction 43) -> Shifting
  (junction 15) -> (junction 20) [order 4] : [commandedGear == GearState.GEAR_PARK]
      | {parkSignal1 = true; parkSignal2 = false;}
  Ready -> (junction 15) : [engaged && (commandedGear ~= currentGear)]
  (junction 15) -> (junction 21) [order 3] : [commandedGear == GearState.GEAR_REVERSE]
      | {signal1 = true; signal2 = true; signal3 = false; signal6 = false;}
  (junction 15) -> (junction 16) [order 1] : [commandedGear == GearState.GEAR_DRIVE || commandedGear == GearState.GEAR_B]
      | {signal3 = false; signal4 = true; signal5 = true; signal6 = false;}
  (junction 21) -> Shifting
  Shifting -> Home : after(1000, tick)
  (junction 16) -> Shifting
  data: engaged input boolean; signal1 output boolean; signal2 output boolean; signal3 output boolean; signal4 output boolean; signal5 output boolean; signal6 output boolean; commandedGear input Enum: GearState; currentGear input Enum: GearState; parkSignal1 output boolean; parkSignal2 output boolean
